simulink model "blance_leg"  (R2023b)
settings: Solver=VariableStepAuto  StartTime=0.0  StopTime=10  MaxStep=0.24  RelTol=1e-3
undefined symbols (not defined in the file or in its folder): k11, k110, k12, k13, k14, k15, k16, k17, k18, k19, k21, k210, k22, k23, k24, k25, k26, k27, k28, k29, k31, k310, k32, k33, k34, k35, k36, k37, k38, k39, k41, k410, k42, k43, k44, k45, k46, k47, k48, k49, X, Y, Z
libraries: sm_lib x114, nesl_utility x23, matrix_library x4, slpidlib x2
(part 4 of 4)

== matlab function blance_leg/Right Controller/MATLAB Function3 ==
  data: d_phi0 output; J input; d_phi1 input; d_phi2 input; d_L0 output
function [d_phi0,d_L0] = D_PHI0(J,d_phi1,d_phi2)
    q_dot = J*[d_phi1;d_phi2];
    d_L0 = q_dot(1);
    d_phi0 = q_dot(2);
    
end

== matlab function blance_leg/MATLAB Function2 ==
  data: phi2_3 output; L0 input
function phi2_3 = PHI2_3(L0)
    l1=0.215;
    l2=0.25;

    phi2_3 = pi - acos((l1*l1+l2*l2-L0*L0)/(2*l1*l2));
end

== matlab function blance_leg/Left Controller/MATLAB Function4 ==
  data: L0 output; phi1 input; phi2 input; phi0 output
function [L0,phi0] = L0_PHI0(phi1,phi2)
    l1=0.15;
    l2=0.25;

    x_C = l1*cos(phi1) + l2*cos(phi2);
    y_C = l1*sin(phi1) + l2*sin(phi2);
    
    L0 = sqrt(x_C*x_C + y_C*y_C);
    phi0 = atan2(y_C,x_C);
end
